simulink model "modellqr1"  (R2023b)
settings: Solver=ode45  StartTime=0.0  StopTime=2500  FixedStep=0.5  RelTol=1e-3
values from neighbouring files (symbols this model uses):
  g_ = 9.81    [main.m]
  h1_ = 0.15    [main.m]
  h2_ = (a^2*h1_)/(b^2)    [main.m]
  K = lqr(A,B,Q,R)    [main.m]
  p1_ = 0.85    [main.m]
  p2_ = 0.95    [main.m]
  q0_ = a*sqrt(h1_)    [main.m]
  s1_ = 0.083    [main.m]
  S1_ = 2*pi*R1_*h1_ + 2*pi*R1_^2    (= 27.0176968209)    [main.m]
  s2_ = 0.083    [main.m]
  S2_ = 2*pi*R2_*h2_ + 2*pi*R2_^2    [main.m]
settings Model: Creator=ralex  LastModifiedBy=ralex

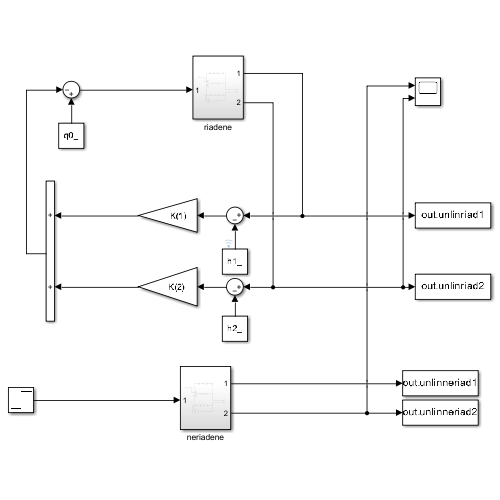
[thumbnail: Simulink's stored preview of the top-level diagram]
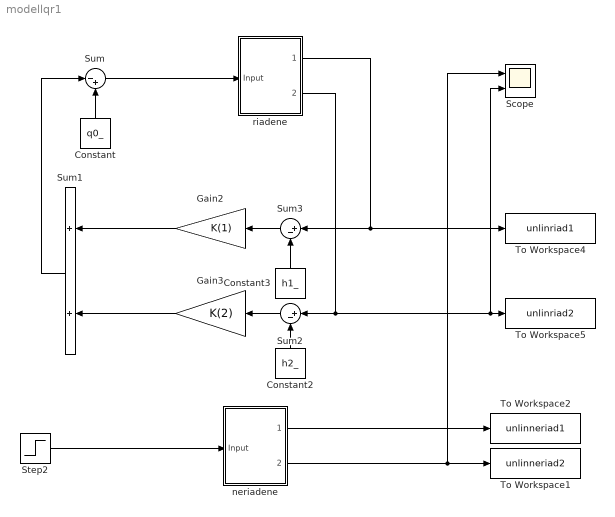
== system modellqr1 ==
  Constant : Constant  Value=q0_
  Constant2 : Constant  Value=h2_
  Constant3 : Constant  Value=h1_
  Gain2 : Gain  Gain=K(1)
  Gain3 : Gain  Gain=K(2)
  Scope : Scope  NumInputPorts=2
  Step2 : Step  Time=1000  Before=q0_  After=q0_  SampleTime=0
  Sum : Sum  Inputs=|-+
  Sum1 : Sum
  Sum2 : Sum  Inputs=|+-
  Sum3 : Sum  Inputs=|+-
  To Workspace1 : ToWorkspace  VariableName=unlinneriad2  SaveFormat=Timeseries  SampleTime=-1
  To Workspace2 : ToWorkspace  VariableName=unlinneriad1  SaveFormat=Timeseries  SampleTime=-1
  To Workspace4 : ToWorkspace  VariableName=unlinriad1  SaveFormat=Timeseries  SampleTime=-1
  To Workspace5 : ToWorkspace  VariableName=unlinriad2  SaveFormat=Timeseries  SampleTime=-1
  neriadene : Subsystem
  riadene : Subsystem
  wires:
  Step2/1 -> neriadene/1(Input)
  neriadene/2(Output) -> Scope/1, To Workspace1/1
  neriadene/1(Output1) -> To Workspace2/1
  Gain3/1 -> Sum1/2
  Gain2/1 -> Sum1/1
  riadene/1(Output1) -> Sum3/1, To Workspace4/1
  Constant3/1 -> Sum3/2
  Constant/1 -> Sum/2
  Sum3/1 -> Gain2/1
  Sum2/1 -> Gain3/1
  Constant2/1 -> Sum2/2
  Sum1/1 -> Sum/1
  riadene/2(Output) -> Scope/2, To Workspace5/1, Sum2/1
  Sum/1 -> riadene/1(Input)

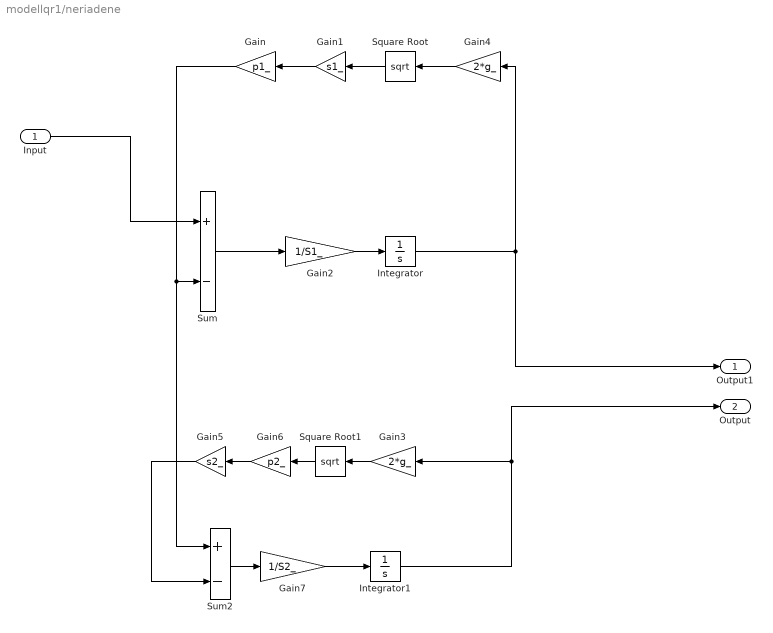
== system modellqr1/neriadene ==
  Input : Inport
  Gain : Gain  Gain=p1_
  Gain1 : Gain  Gain=s1_
  Gain2 : Gain  Gain=1/S1_
  Gain3 : Gain  Gain=2*g_
  Gain4 : Gain  Gain=2*g_
  Gain5 : Gain  Gain=s2_
  Gain6 : Gain  Gain=p2_
  Gain7 : Gain  Gain=1/S2_
  Integrator : Integrator  InitialCondition=h1_-h1_/5
  Integrator1 : Integrator  InitialCondition=h2_-h2_/5
  Square Root : Sqrt
  Square Root1 : Sqrt
  Sum : Sum  Inputs=+-
  Sum2 : Sum  Inputs=+-
  Output1 : Outport
  Output : Outport  Port=2
  wires:
  Gain/1 -> Sum/2, Sum2/1
  Gain1/1 -> Gain/1
  Input/1 -> Sum/1
  Integrator/1 -> Output1/1, Gain4/1
  Square Root/1 -> Gain1/1
  Gain4/1 -> Square Root/1
  Gain5/1 -> Sum2/2
  Sum/1 -> Gain2/1
  Integrator1/1 -> Output/1, Gain3/1
  Gain6/1 -> Gain5/1
  Square Root1/1 -> Gain6/1
  Gain3/1 -> Square Root1/1
  Sum2/1 -> Gain7/1
  Gain2/1 -> Integrator/1
  Gain7/1 -> Integrator1/1

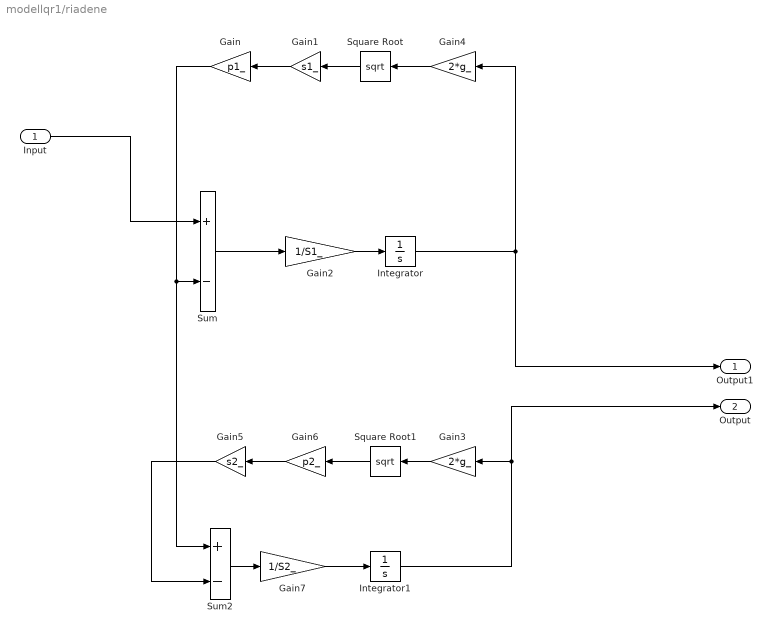
== system modellqr1/riadene ==
  Input : Inport
  Gain : Gain  Gain=p1_
  Gain1 : Gain  Gain=s1_
  Gain2 : Gain  Gain=1/S1_
  Gain3 : Gain  Gain=2*g_
  Gain4 : Gain  Gain=2*g_
  Gain5 : Gain  Gain=s2_
  Gain6 : Gain  Gain=p2_
  Gain7 : Gain  Gain=1/S2_
  Integrator : Integrator  InitialCondition=h1_-h1_/5
  Integrator1 : Integrator  InitialCondition=h2_-h2_/5
  Square Root : Sqrt
  Square Root1 : Sqrt
  Sum : Sum  Inputs=+-
  Sum2 : Sum  Inputs=+-
  Output1 : Outport
  Output : Outport  Port=2
  wires:
  Gain/1 -> Sum/2, Sum2/1
  Gain1/1 -> Gain/1
  Input/1 -> Sum/1
  Integrator/1 -> Output1/1, Gain4/1
  Square Root/1 -> Gain1/1
  Gain4/1 -> Square Root/1
  Gain5/1 -> Sum2/2
  Sum/1 -> Gain2/1
  Integrator1/1 -> Output/1, Gain3/1
  Gain6/1 -> Gain5/1
  Square Root1/1 -> Gain6/1
  Gain3/1 -> Square Root1/1
  Sum2/1 -> Gain7/1
  Gain2/1 -> Integrator/1
  Gain7/1 -> Integrator1/1
